simulink model "gyroscope_sim"  (R2023b)
settings: Solver=VariableStepAuto  StartTime=0.0  StopTime=100  RelTol=1e-3
libraries: eeGeneralControl x3
settings Model: NumberOfSteps=5  Creator=jevin  LastModifiedBy=jevin

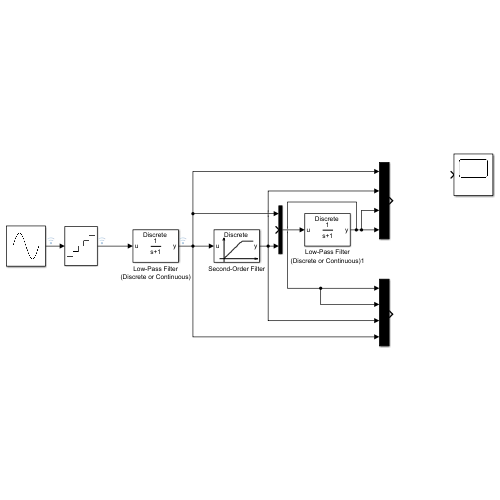
[thumbnail: Simulink's stored preview of the top-level diagram]
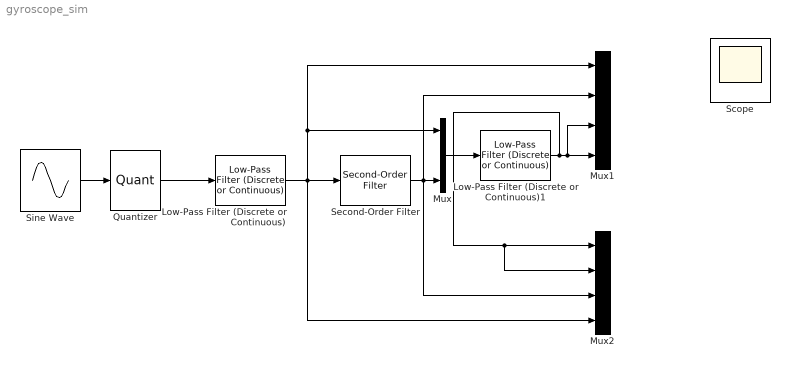
== system gyroscope_sim ==
  Low-Pass Filter (Discrete or Continuous) : eeGeneralControl/Low-Pass Filter (Discrete or Continuous)  K=1  T=1  B=0.8  A=-0.8  init_option=Inherited from block input  x0=1  Ts=-1
  Low-Pass Filter (Discrete or Continuous)1 : eeGeneralControl/Low-Pass Filter (Discrete or Continuous)  K=1  T=1  B=inf  A=-inf  init_option=Inherited from block input  x0=0  Ts=-1
  Mux : Mux  Inputs=3
  Mux1 : Mux
  Mux2 : Mux
  Quantizer : Quantizer
  Scope : Scope
  Second-Order Filter : eeGeneralControl/Second-Order Filter  FilterType=High-pass  fn=60  Zeta=0.707  Ts=-1  A0=0.5  Ph0=0.5  f0=0.5  b0=0.5
      settings: LibrarySourceBlock=ee_sl_lib/General Control/Second-Order Filter
  Sine Wave : Sin  SampleTime=0
  wires:
  Sine Wave/1 -> Quantizer/1
  Quantizer/1 -> Low-Pass Filter (Discrete or Continuous)/1
  Mux/1 -> Low-Pass Filter (Discrete or Continuous)1/1
  Second-Order Filter/1 -> Mux2/3, Mux1/2, Mux/3
  Low-Pass Filter (Discrete or Continuous)/1 -> Second-Order Filter/1, Mux2/4, Mux1/1, Mux/1
  Low-Pass Filter (Discrete or Continuous)1/1 -> Mux2/2, Mux2/1, Mux1/3, Mux1/4
